simulink model "ERLE"  (R2013a)
settings: Solver=FixedStepDiscrete  StartTime=0.0  StopTime=10.0  RelTol=1e-3
values from neighbouring files (symbols this model uses):
  M = 0.95    [Variaveis.mat]
settings Model: Creator=Élio  LastModifiedBy=Élio

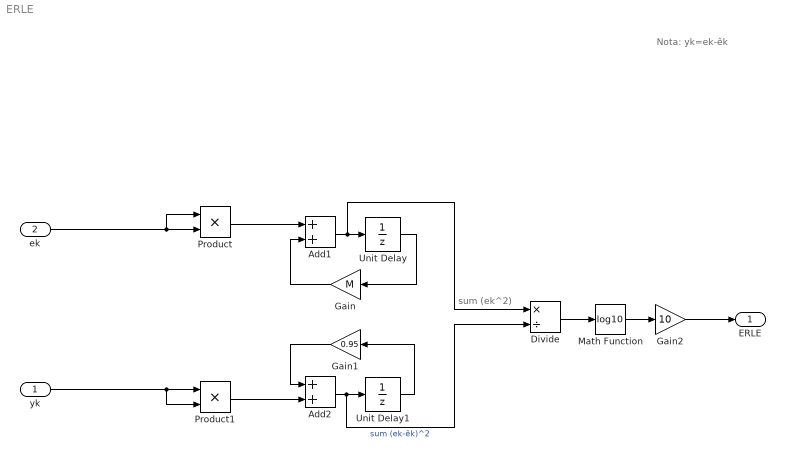
== system ERLE ==
  note: Nota: yk=ek-êk
  note: sum (ek^2)
  yk : Inport
  ek : Inport  Port=2
  Add1 : Sum  RequirementInfo={} %GIDa_2cfc2820_417e_4e29_b3e1_8803327010a5
  Add2 : Sum  RequirementInfo={} %GIDa_0975e0af_af49_4f1e_9480_dc816cb5e02c
  Divide : Product  Inputs=*/
  Gain : Gain  Gain=M  SampleTime=M
  Gain1 : Gain  Gain=0.95
  Gain2 : Gain  Gain=10
  Math Function : Math  Operator=log10  SaturateOnIntegerOverflow=on
  Product : Product
  Product1 : Product
  Unit Delay : UnitDelay  SampleTime=-1
  Unit Delay1 : UnitDelay  SampleTime=-1
  ERLE : Outport
  wires:
  yk/1 -> Product1/2, Product1/1
  Math Function/1 -> Gain2/1
  Add2/1 -> Divide/2, Unit Delay1/1  "sum (ek-êk)^2"
  Product/1 -> Add1/1
  Gain1/1 -> Add2/1
  Divide/1 -> Math Function/1
  Gain2/1 -> ERLE/1
  Unit Delay1/1 -> Gain1/1
  Add1/1 -> Divide/1, Unit Delay/1
  Unit Delay/1 -> Gain/1
  ek/1 -> Product/2, Product/1
  Gain/1 -> Add1/2
  Product1/1 -> Add2/2
